simulink model "system"  (R2019b)
settings: Solver=VariableStepAuto  StartTime=0.0  StopTime=10.0  RelTol=1e-3
values from neighbouring files (symbols this model uses):
  k_1 = 8    [Labs2.m]
  k_4 = 8    [Labs2.m]
  T_2 = 2    [Labs2.m]
  T_31 = 2    [Labs2.m]
  T_32 = 3    [Labs2.m]
  tau_2 = 3    [Labs2.m]
  zetta_31 = 0.75    [Labs2.m]
  zetta_32 = 0.5    [Labs2.m]
settings Model: Creator=Danya  LastModifiedBy=Danya

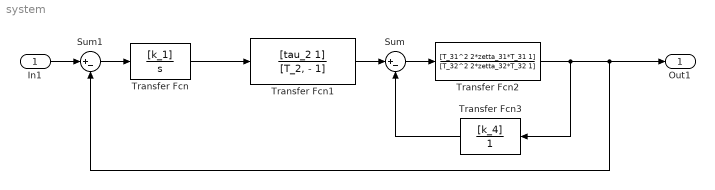
== system system ==
  In1 : Inport
  Sum : Sum  Inputs=|+-
  Sum1 : Sum  Inputs=|+-
  Transfer Fcn : TransferFcn  Numerator=[k_1]  Denominator=[1 0]
  Transfer Fcn1 : TransferFcn  Numerator=[tau_2 1]  Denominator=[T_2, - 1]
  Transfer Fcn2 : TransferFcn  Numerator=[T_31^2 2*zetta_31*T_31 1]  Denominator=[T_32^2 2*zetta_32*T_32 1]
  Transfer Fcn3 : TransferFcn  Numerator=[k_4]  Denominator=[1]
  Out1 : Outport
  wires:
  Transfer Fcn/1 -> Transfer Fcn1/1
  Transfer Fcn1/1 -> Sum/1
  Sum/1 -> Transfer Fcn2/1
  Transfer Fcn2/1 -> Transfer Fcn3/1, Out1/1, Sum1/2
  Transfer Fcn3/1 -> Sum/2
  Sum1/1 -> Transfer Fcn/1
  In1/1 -> Sum1/1
